simulink model "Stability"  (R2022b)
settings: Solver=VariableStepAuto  StartTime=0.0  StopTime=60  RelTol=1e-3
settings Model: Creator=eder  LastModifiedBy=eder

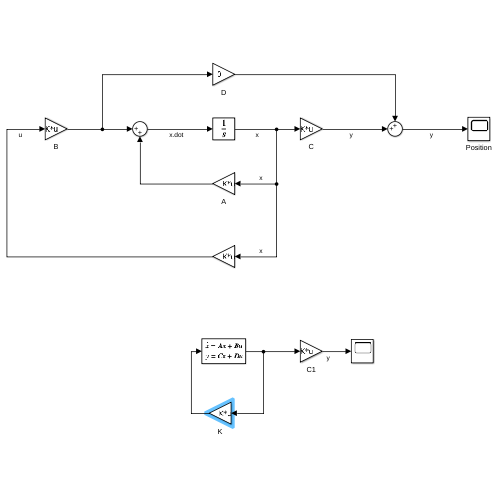
[thumbnail: Simulink's stored preview of the top-level diagram]
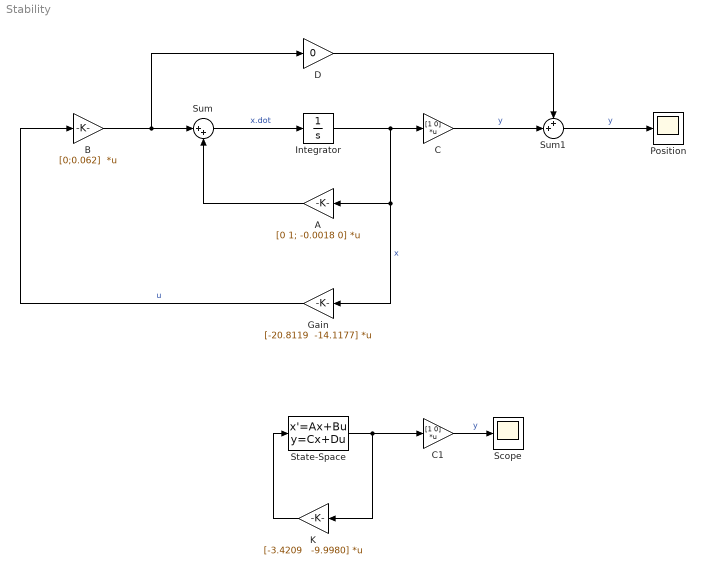
== system Stability ==
  A : Gain  Gain=[0 1; -0.0018 0]  Multiplication=Matrix(K*u)
  B : Gain  Gain=[0;0.062]  Multiplication=Matrix(K*u)
  C : Gain  Gain=[1 0]  Multiplication=Matrix(K*u)
  C1 : Gain  Gain=[1 0]  Multiplication=Matrix(K*u)
  D : Gain  Gain=0
  Gain : Gain  Gain="[-20.8119  -14.1177]"  Multiplication=Matrix(K*u)
  Integrator : Integrator  InitialCondition=[-pi*.3;0]
  K : Gain  Gain="[-3.4209   -9.9980]"  Multiplication=Matrix(K*u)
  Position : Scope
  Scope : Scope
  State-Space : StateSpace  A=[0 1; -0.0018 0]  B=[0;0.062]  C=[1 0;0 1]  D=[0;0]  InitialCondition=[-pi*.3;0]
  Sum : Sum  Inputs=|++
  Sum1 : Sum  Inputs=++|
  wires:
  State-Space/1 -> C1/1, K/1
  K/1 -> State-Space/1
  C/1 -> Sum1/2  "y"
  D/1 -> Sum1/1
  A/1 -> Sum/2
  Sum/1 -> Integrator/1  "x.dot"
  Sum1/1 -> Position/1  "y"
  C1/1 -> Scope/1  "y"
  Gain/1 -> B/1  "u"
  Integrator/1 -> A/1, Gain/1, C/1  "x"
  B/1 -> D/1, Sum/1
